simulink model "ReqTableTest"  (R2022b)
settings: Solver=VariableStepAuto  StartTime=0.0  StopTime=10.0  RelTol=1e-3
settings Model: Creator=fedformi_new  LastModifiedBy=ChrisGeorge

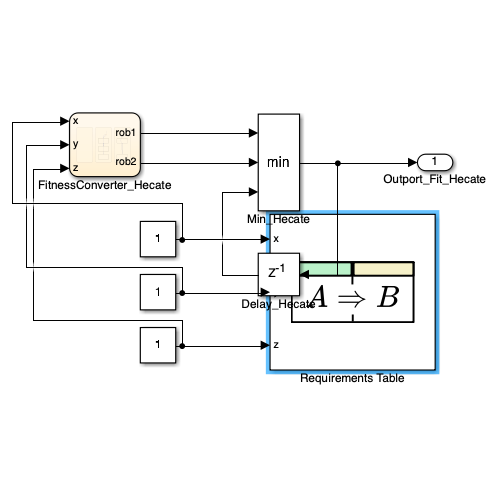
[thumbnail: Simulink's stored preview of the top-level diagram]
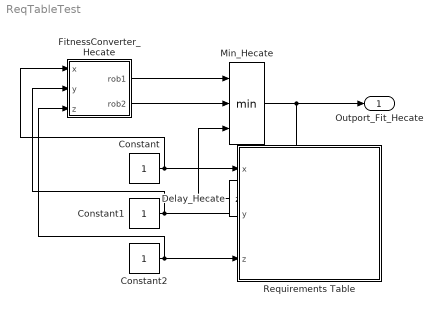
== system ReqTableTest ==
  Constant : Constant
  Constant1 : Constant
  Constant2 : Constant
  Delay_Hecate : Delay  DelayLength=1  InitialCondition=Inf
  FitnessConverter_Hecate : Stateflow chart  TreatAsAtomicUnit=on
  Min_Hecate : MinMax  Inputs=3
  Requirements Table : Requirements Table  TreatAsAtomicUnit=on
  Outport_Fit_Hecate : Outport
  wires:
  Constant/1 -> Requirements Table/1(x), FitnessConverter_Hecate/1(x)
  Constant1/1 -> Requirements Table/2(y), FitnessConverter_Hecate/2(y)
  Constant2/1 -> Requirements Table/3(z), FitnessConverter_Hecate/3(z)
  FitnessConverter_Hecate/1(rob1) -> Min_Hecate/1
  FitnessConverter_Hecate/2(rob2) -> Min_Hecate/2
  Min_Hecate/1 -> Delay_Hecate/1, Outport_Fit_Hecate/1
  Delay_Hecate/1 -> Min_Hecate/3

== stateflow chart ReqTableTest/FitnessConverter_Hecate ==
  state Assumptions_check [parallel]
    assert((~(y < 0) || (y < 0 && x > 2)) && (~(y >= 2) || (y >= 2 && x > 5)) && (~(y < 0 && x < -3) || (y < 0 && x < -3 && y < -7)),"One of the model assumptions have been violated.");
    settings: executionOrder=1
  state Requirement_1 [parallel]
    settings: executionOrder=2
    state Default
      rob1 = Inf;
    state Wait
      rob1 = Inf;
    state Verify
      rob1 = (z-(1));
    (default) -> (junction 8)
    (junction 8) -> Wait [order 2]
    (junction 8) -> Requirement_1.Default [order 1] : [~((x>0) && (y>0))]
    Requirement_1.Default -> Wait : [(x>0) && (y>0)]
    Wait -> Requirement_1.Default [order 1] : [~((x>0) && (y>0))]
    Requirement_1.Verify -> Requirement_1.Default : [~((x>0) && (y>0))]
    Wait -> Requirement_1.Verify [order 2] : [et >= 5]
  state Requirement_2 [parallel]
    settings: executionOrder=3
    state Default
      rob2 = Inf;
    state Verify
      rob2 = (abs(z)-(1));
    (default) -> (junction 20)
    (junction 20) -> Requirement_2.Verify [order 2]
    (junction 20) -> Requirement_2.Default [order 1] : [~((abs(x)>0) && (abs(y)>0))]
    Requirement_2.Default -> Requirement_2.Verify : [(abs(x)>0) && (abs(y)>0)]
    Requirement_2.Verify -> Requirement_2.Default : [~((abs(x)>0) && (abs(y)>0))]
  data: x input; y input; z input; rob1 output double =Inf; rob2 output double =Inf

== stateflow chart ReqTableTest/Requirements Table ==
  (default) -> (junction 1073745165)
  (junction 1073745165) -> (junction 1073745166) : {
      | % SF_REQ_REV_07
      | }
  (junction 1073745166) -> (junction 1073745168) : {
      | % HEADER_ASSIGNMENTS
      |
      | }
  (junction 1073745168) -> (junction 1073745170) : {
      | % START_A_4
      | }
  (junction 1073745170) -> (junction 1073745172) : {
      | }
  (junction 1073745172) -> (junction 1073745174)
  (junction 1073745174) -> (junction 1073745176) [order 1] : [(y < 0)]
  (junction 1073745174) -> (junction 1073745200) [order 2]
  (junction 1073745176) -> (junction 1073745178) : {
      | reqtable_assumption((x > 2), 4);
      | }
  (junction 1073745178) -> (junction 1073745180) : {
      | }
  (junction 1073745180) -> (junction 1073745182) : {
      | % START_A_7
      | }
  (junction 1073745182) -> (junction 1073745184) : {
      | }
  (junction 1073745184) -> (junction 1073745186)
  (junction 1073745186) -> (junction 1073745188) [order 1] : [(x < -3)]
  (junction 1073745186) -> (junction 1073745194) [order 2]
  (junction 1073745188) -> (junction 1073745190) : {
      | reqtable_assumption((y < -7), 7);
      | }
  (junction 1073745190) -> (junction 1073745192) : {
      | }
  (junction 1073745192) -> (junction 1073745194)
  (junction 1073745194) -> (junction 1073745196)
  (junction 1073745196) -> (junction 1073745198) : {
      | % END_A_7
      | }
  (junction 1073745198) -> (junction 1073745200)
  (junction 1073745200) -> (junction 1073745202)
  (junction 1073745202) -> (junction 1073745204) : {
      | % END_A_4
      | }
  (junction 1073745204) -> (junction 1073745206) : {
      | % START_A_28
      | }
  (junction 1073745206) -> (junction 1073745208) : {
      | }
  (junction 1073745208) -> (junction 1073745210)
  (junction 1073745210) -> (junction 1073745212) [order 1] : [(y >= 2)]
  (junction 1073745210) -> (junction 1073745218) [order 2]
  (junction 1073745212) -> (junction 1073745214) : {
      | reqtable_assumption((x > 5), 28);
      | }
  (junction 1073745214) -> (junction 1073745216) : {
      | }
  (junction 1073745216) -> (junction 1073745218)
  (junction 1073745218) -> (junction 1073745220)
  (junction 1073745220) -> (junction 1073745599) : {
      | % END_A_28
      | }
  (junction 1073745599) -> (junction 1073745358) : {
      | % START_R_1
      | }
  (junction 1073745358) -> (junction 1073745360) : {
      | }
  (junction 1073745360) -> (junction 1073745362)
  (junction 1073745362) -> (junction 1073745364) [order 1] : [duration(((x) > 0) && ((y) > 0)) >= 5]
  (junction 1073745362) -> (junction 1073745370) [order 2]
  (junction 1073745364) -> (junction 1073745366) : {
      | reqtable_postcondition((z > 1), 'R:1');
      |
      |
      | }
  (junction 1073745366) -> (junction 1073745368) : {
      | }
  (junction 1073745368) -> (junction 1073745370)
  (junction 1073745370) -> (junction 1073745372)
  (junction 1073745372) -> (junction 1073745428) : {
      | % END_R_1
      | }
  (junction 1073745428) -> (junction 1073745692) : {
      | % START_R_46
      | }
  (junction 1073745692) -> (junction 1073745694) : {
      | }
  (junction 1073745694) -> (junction 1073745696)
  (junction 1073745696) -> (junction 1073745698) [order 1] : [(abs((x)) > 0) && (abs((y)) > 0)]
  (junction 1073745696) -> (junction 1073745704) [order 2]
  (junction 1073745698) -> (junction 1073745700) : {
      | reqtable_postcondition((abs(z) > 1), 'R:2');
      |
      |
      | }
  (junction 1073745700) -> (junction 1073745702) : {
      | }
  (junction 1073745702) -> (junction 1073745704)
  (junction 1073745704) -> (junction 1073745706)
  (junction 1073745706) -> (junction 1073745708) : {
      | % END_R_46
      | }
  data: x input; y input; z input
